simulink model "ceti_b4_xx_transimpedance_linearization"  (R2023a)
settings: Solver=FixedStepAuto  StartTime=0.0  StopTime=0.05  FixedStep=0.0001  RelTol=1e-3
settings Model: Creator=Villou  LastModifiedBy=Villou

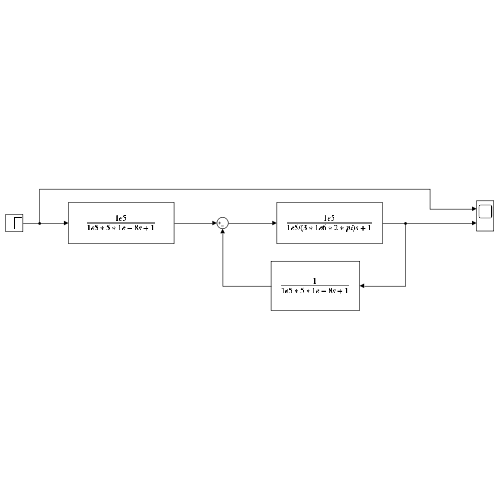
[thumbnail: Simulink's stored preview of the top-level diagram]
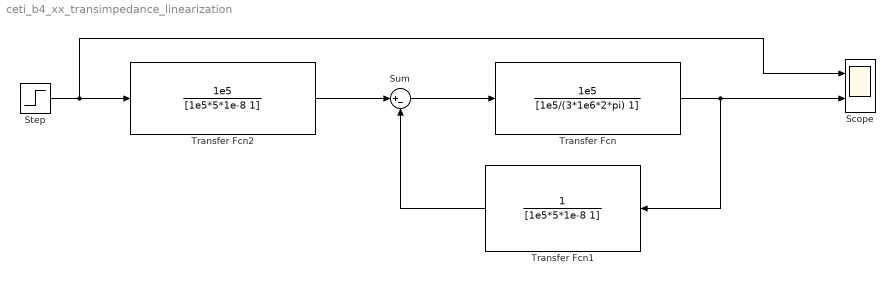
== system ceti_b4_xx_transimpedance_linearization ==
  Scope : Scope  NumInputPorts=2
  Step : Step  Time=0.01  SampleTime=0
  Sum : Sum  Inputs=|+-
  Transfer Fcn : TransferFcn  Numerator=[1e5]  Denominator=[1e5/(3*1e6*2*pi) 1]
  Transfer Fcn1 : TransferFcn  Denominator=[1e5*5*1e-8 1]
  Transfer Fcn2 : TransferFcn  Numerator=[1e5]  Denominator=[1e5*5*1e-8 1]
  wires:
  Sum/1 -> Transfer Fcn/1
  Transfer Fcn1/1 -> Sum/2
  Transfer Fcn/1 -> Scope/2, Transfer Fcn1/1
  Transfer Fcn2/1 -> Sum/1
  Step/1 -> Scope/1, Transfer Fcn2/1
